simulink model "CSTR"  (R2020a)
settings: Solver=VariableStepAuto  StartTime=0.0  StopTime=15  MaxStep=10e-3  RelTol=1e-3
values from neighbouring files (symbols this model uses):
  Ca0 = 2.917496611031752    (= 2.91749661103)    [CSTRComputeOP.m]    (also in CSTRInit.m)
  Cb0 = 1.099991103606458    (= 1.09999110361)    [CSTRComputeOP.m]    (also in CSTRInit.m)
  k1 = 5/6    (= 0.833333333333)    [CSTRComputeOP.m]    (also in CSTRInit.m; CSTROP.m = param(1); sfun_CSTR.m = param(1))
  k2 = 5/3    (= 1.66666666667)    [CSTRComputeOP.m]    (also in CSTRInit.m; CSTROP.m = param(2); sfun_CSTR.m = param(2))
  k3 = 1/6    (= 0.166666666667)    [CSTRComputeOP.m]    (also in CSTRInit.m; CSTROP.m = param(3); sfun_CSTR.m = param(3))
  V = 700    [CSTRComputeOP.m]    (also in CSTRInit.m; CSTROP.m = param(4); sfun_CSTR.m = param(4))
settings Model: Creator=david  LastModifiedBy=david

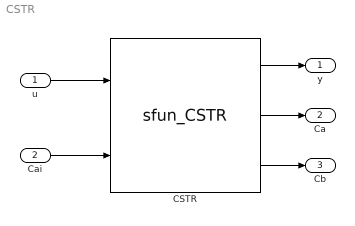
== system CSTR ==
  u : Inport
  Cai : Inport  Port=2
  CSTR : M-S-Function  FunctionName=sfun_CSTR  Parameters=|  mask{k1=k1, k2=k2, k3=k3, V=V, Ca0=Ca0, Cb0=Cb0}
      | [k1;
      | k2;
      | k3; V], [Ca0; Cb0]
      mask DialogControl DescGroupVar Prompt: Isothermal Van de Vusse reactor
      mask DialogControl DescTextVar Prompt: Model for the isothermal Van de Vusse reaction in a CSTR with constant volume
      mask Display:
      | port_label('output', 1, 'y')
      | port_label('output', 2, 'Ca')
      | port_label('output', 3, 'Cb')
      | port_label('input', 1, 'u')
      | port_label('input', 2, 'Cai')
      | image('VandeVusse.png')
  y : Outport
  Ca : Outport  Port=2
  Cb : Outport  Port=3
  wires:
  u/1 -> CSTR/1
  Cai/1 -> CSTR/2
  CSTR/1 -> y/1
  CSTR/2 -> Ca/1
  CSTR/3 -> Cb/1
